simulink model "echo4"  (R2020b)
settings: Solver=VariableStepAuto  StartTime=0.0  StopTime=stop_time  RelTol=1e-3
InitFcn:
  | callback_init
StopFcn:
  | callback_stop
undefined symbols (not defined in the file or in its folder): mp
libraries: simulink x1, hdlsllib x1
settings Model: Creator=mvale_7a44q92  LastModifiedBy=mvale_7a44q92
settings DataIOCC: ReturnWorkspaceOutputs=off

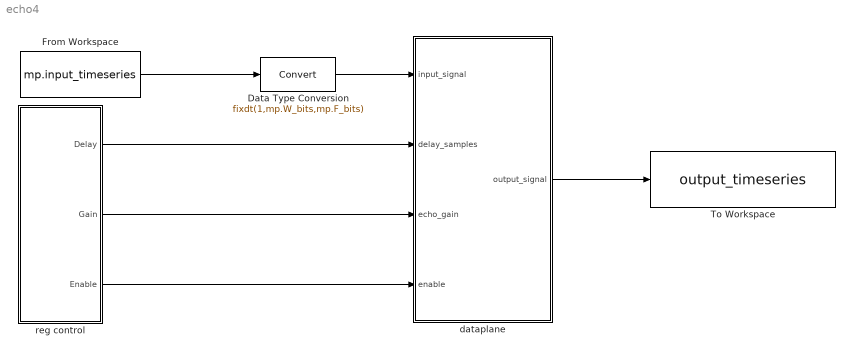
== system echo4 ==
  Data Type Conversion : DataTypeConversion  OutDataTypeStr=fixdt(1,mp.W_bits,mp.F_bits)
  From Workspace : FromWorkspace  VariableName=mp.input_timeseries  SampleTime=mp.Ts  OutputAfterFinalValue=Holding final value
  To Workspace : ToWorkspace  VariableName=output_timeseries  SaveFormat=Timeseries  SampleTime=-1
  dataplane : Subsystem
  reg control : Subsystem
  wires:
  From Workspace/1 -> Data Type Conversion/1
  dataplane/1(output_signal) -> To Workspace/1
  reg control/1(Delay) -> dataplane/2(delay_samples)
  reg control/2(Gain) -> dataplane/3(echo_gain)
  reg control/3(Enable) -> dataplane/4(enable)
  Data Type Conversion/1 -> dataplane/1(input_signal)

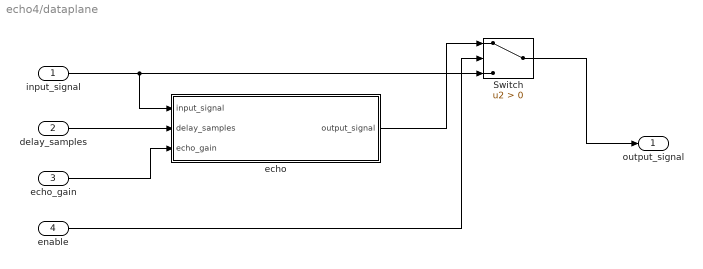
== system echo4/dataplane ==
  input_signal : Inport
  delay_samples : Inport  Port=2
  echo_gain : Inport  Port=3
  enable : Inport  Port=4
  Switch : Switch  Criteria=u2 > Threshold
  echo : Subsystem
  output_signal : Outport
  wires:
  input_signal/1 -> echo/1(input_signal), Switch/3
  echo/1(output_signal) -> Switch/1
  delay_samples/1 -> echo/2(delay_samples)
  enable/1 -> Switch/2
  echo_gain/1 -> echo/3(echo_gain)
  Switch/1 -> output_signal/1

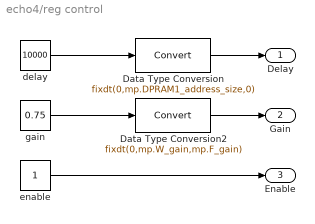
== system echo4/reg control ==
  Data Type Conversion : DataTypeConversion  OutDataTypeStr=fixdt(0,mp.DPRAM1_address_size,0)
  Data Type Conversion2 : DataTypeConversion  OutDataTypeStr=fixdt(0,mp.W_gain,mp.F_gain)
  delay : Constant  Value=10000  SampleTime=mp.Ts
  enable : Constant  OutDataTypeStr=boolean  SampleTime=mp.Ts
  gain : Constant  Value=0.75  SampleTime=mp.Ts
  Delay : Outport
  Gain : Outport  Port=2
  Enable : Outport  Port=3
  wires:
  delay/1 -> Data Type Conversion/1
  enable/1 -> Enable/1
  Data Type Conversion/1 -> Delay/1
  gain/1 -> Data Type Conversion2/1
  Data Type Conversion2/1 -> Gain/1

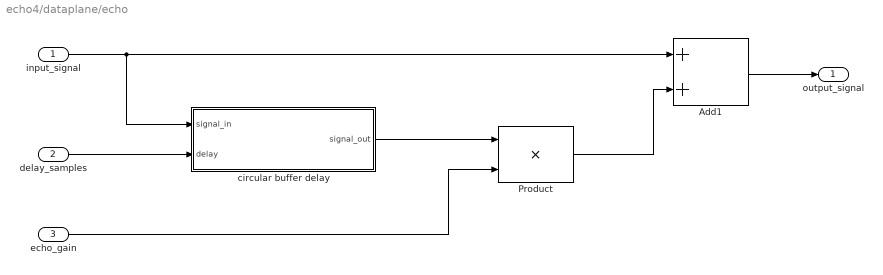
== system echo4/dataplane/echo ==
  input_signal : Inport
  delay_samples : Inport  Port=2
  echo_gain : Inport  Port=3
  Add1 : Sum  OutDataTypeStr=Inherit: Same as first input
  Product : Product  OutDataTypeStr=Inherit: Same as first input
  circular buffer delay : Subsystem
  output_signal : Outport
  wires:
  Add1/1 -> output_signal/1
  input_signal/1 -> circular buffer delay/1(signal_in), Add1/1
  Product/1 -> Add1/2
  echo_gain/1 -> Product/2
  delay_samples/1 -> circular buffer delay/2(delay)
  circular buffer delay/1(signal_out) -> Product/1

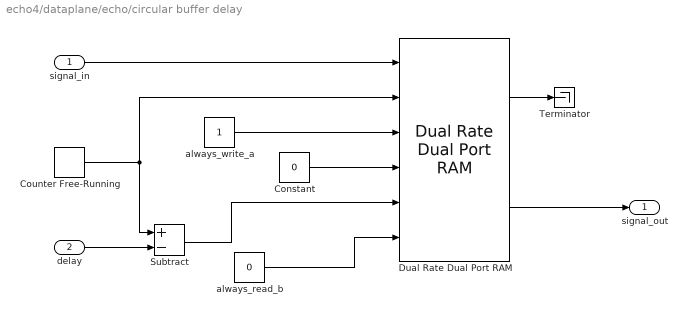
== system echo4/dataplane/echo/circular buffer delay ==
  signal_in : Inport
  delay : Inport  Port=2
  Constant : Constant  Value=0  OutDataTypeStr=fixdt(1,mp.W_bits,mp.F_bits)  SampleTime=mp.Ts
  Counter Free-Running : simulink/Sources/Counter Free-Running  NumBits=mp.DPRAM1_address_size  tsamp=mp.Ts
  Dual Rate Dual Port RAM : hdlsllib/HDL RAMs/Dual Rate Dual Port RAM  ram_size=mp.DPRAM1_address_size
      settings: SourceProductBaseCode=SL
  Subtract : Sum  Inputs=+-  OutDataTypeStr=Inherit: Same as first input
  Terminator : Terminator
  always_read_b : Constant  Value=0  OutDataTypeStr=boolean  SampleTime=mp.Ts
  always_write_a : Constant  OutDataTypeStr=boolean  SampleTime=mp.Ts
  signal_out : Outport
  wires:
  Subtract/1 -> Dual Rate Dual Port RAM/5
  signal_in/1 -> Dual Rate Dual Port RAM/1
  Constant/1 -> Dual Rate Dual Port RAM/4
  Counter Free-Running/1 -> Subtract/1, Dual Rate Dual Port RAM/2
  Dual Rate Dual Port RAM/2 -> signal_out/1
  always_write_a/1 -> Dual Rate Dual Port RAM/3
  always_read_b/1 -> Dual Rate Dual Port RAM/6
  delay/1 -> Subtract/2
  Dual Rate Dual Port RAM/1 -> Terminator/1
